simulink model "EE563TermProjectErencanDuymaz"  (R2013a)
settings: Solver=ode4  StartTime=0.0  StopTime=2  FixedStep=1/25600  RelTol=1e-3
libraries: powerlib_meascontrol x44, simulink x8, powerlib x1
settings Model: Creator=Eren  LastModifiedBy=Eren

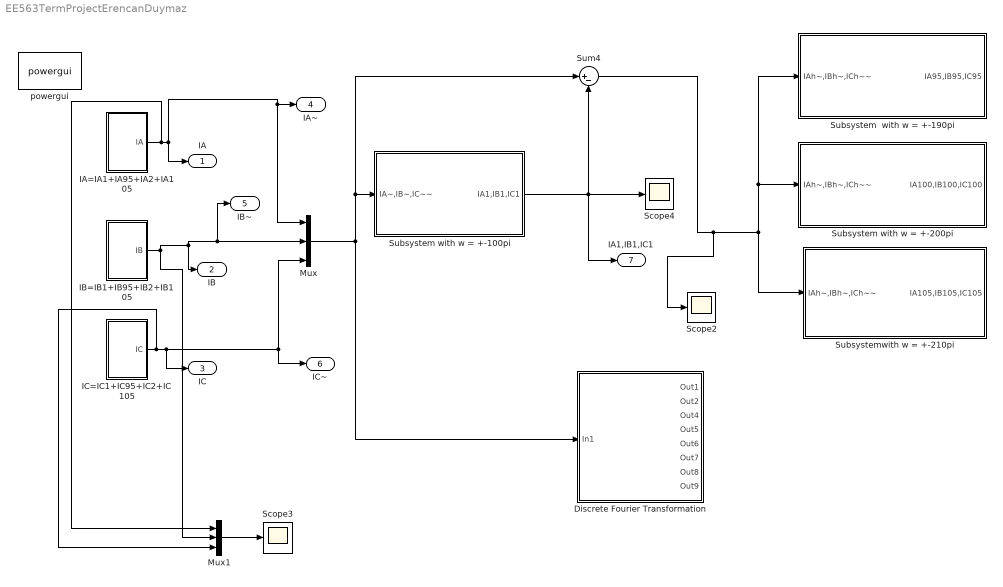
== system EE563TermProjectErencanDuymaz ==
  Discrete Fourier Transformation : Subsystem
  "IA=IA1+IA95+IA2+IA105 " : Subsystem
  "IB=IB1+IB95+IB2+IB105 " : Subsystem
  "IC=IC1+IC95+IC2+IC105 " : Subsystem
  Mux : Mux  Inputs=3
  Mux1 : Mux  Inputs=3
  Scope2 : Scope
      settings: YMin=-1000  YMax=1000  SaveName=ScopeData5
  Scope3 : Scope
      settings: TimeRange=0.2005801931657021  YMin=-3000  YMax=3000  SaveName=ScopeData8
  Scope4 : Scope
      settings: YMin=-3000  YMax=3000  SaveName=ScopeData7
  Subsystem  with w = +-190pi : Subsystem
  Subsystem with w = +-100pi : Subsystem
  Subsystem with w = +-200pi : Subsystem
  "Subsystemwith w = +-210pi " : Subsystem
  Sum4 : Sum  Inputs=|+-
  powergui : powerlib/powergui  Priority=1  SimulationMode=Continuous  SolverType=Tustin  SampleTime=50e-6  frequency=60  SPID=off  DisableSnubberDevices=off  DisableRonSwitches=off  DisableVfSwitches=off  SwTol=0  Interpol=off  DisplayEquations=off  frequencyindice=50  Pbase=100e6  ErrMax=1e-4  Iterations=50  UnitsV=kV  UnitsW=MW  FunctionMessages=off  echomessages=off  HookPort=off  EnableUseOfTLC=off  x0status=blocks  RestoreLinks=warning  ResistiveCurrentMeasurement=off  Frange=[0:2:500]  Ylog=off  Xlog=on  ShowGrid=off  save=off  variable=ZData  ZoomFFT=off  StartTime=0.0  cycles=1  DisplayStyle=1  fundamental=60  FreqAxis=off  MaxFrequency=1000  frequencyindicesteady=1  RmsSteady=1  display=off  Ts=0  methode=off
  IA : Outport
  "IB " : Outport  Port=2
  "IC " : Outport  Port=3
  "IA~ " : Outport  Port=4
  IB~ : Outport  Port=5
  IC~ : Outport  Port=6
  IA1,IB1,IC1 : Outport  Port=7
  wires:
  "IA=IA1+IA95+IA2+IA105 "/1(IA) -> Mux1/1, Mux/1, "IA~ "/1, IA/1
  "IB=IB1+IB95+IB2+IB105 "/1("IB ") -> Mux/2, IB~/1, "IB "/1, Mux1/2
  "IC=IC1+IC95+IC2+IC105 "/1("IC ") -> Mux1/3, "IC "/1, Mux/3, IC~/1
  Mux/1 -> Sum4/1, Subsystem with w = +-100pi/1(IA~,IB~,IC~~), Discrete Fourier Transformation/1(In1)
  Subsystem with w = +-100pi/1(IA1,IB1,IC1) -> Scope4/1, IA1,IB1,IC1/1, Sum4/2
  Sum4/1 -> Subsystem  with w = +-190pi/1(IAh~,IBh~,ICh~~), Subsystem with w = +-200pi/1(IAh~,IBh~,ICh~~), "Subsystemwith w = +-210pi "/1(IAh~,IBh~,ICh~~), Scope2/1
  Mux1/1 -> Scope3/1

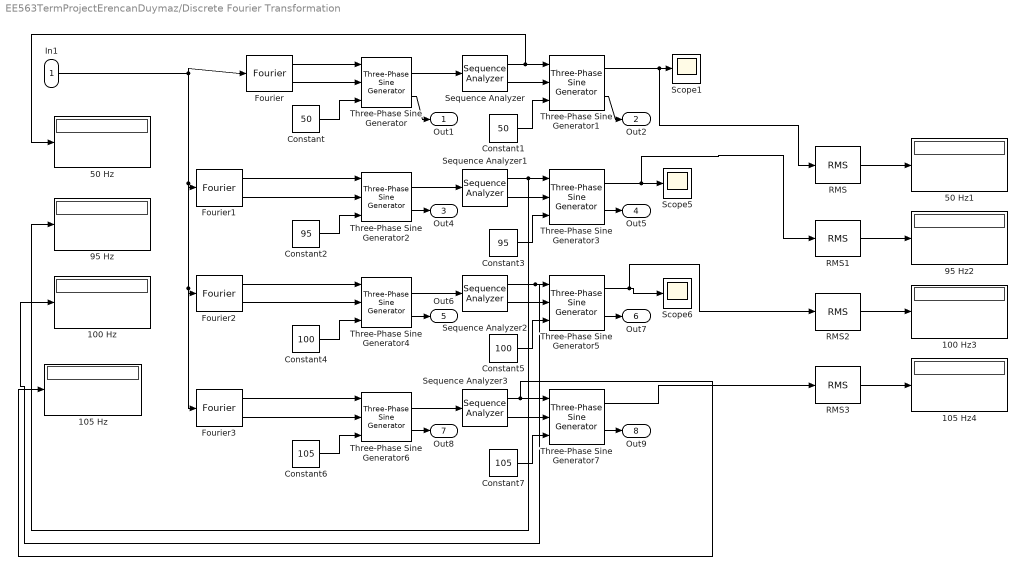
== system EE563TermProjectErencanDuymaz/Discrete Fourier Transformation ==
  In1 : Inport
  100 Hz : Display
  100 Hz3 : Display
  105 Hz : Display
  105 Hz4 : Display
  50 Hz : Display
  50 Hz1 : Display
  "95 Hz " : Display
  95 Hz2 : Display
  Constant : Constant  Value=50
  Constant1 : Constant  Value=50
  Constant2 : Constant  Value=95
  Constant3 : Constant  Value=95
  Constant4 : Constant  Value=100
  Constant5 : Constant  Value=100
  Constant6 : Constant  Value=105
  Constant7 : Constant  Value=105
  Fourier : powerlib_meascontrol/Measurements/Fourier  Freq=5  n=10  InInit=[0, 0]  Ts=0
  Fourier1 : powerlib_meascontrol/Measurements/Fourier  Freq=5  n=19  InInit=[0, 0]  Ts=0
  Fourier2 : powerlib_meascontrol/Measurements/Fourier  Freq=5  n=20  InInit=[0, 0]  Ts=0
  Fourier3 : powerlib_meascontrol/Measurements/Fourier  Freq=5  n=21  InInit=[0, 0]  Ts=0
  RMS : powerlib_meascontrol/Measurements/RMS  TrueRMS=on  Freq=50  RMSInit=120  Ts=0
  RMS1 : powerlib_meascontrol/Measurements/RMS  TrueRMS=on  Freq=95  RMSInit=120  Ts=0
  RMS2 : powerlib_meascontrol/Measurements/RMS  TrueRMS=on  Freq=100  RMSInit=120  Ts=0
  RMS3 : powerlib_meascontrol/Measurements/RMS  TrueRMS=on  Freq=105  RMSInit=120  Ts=0
  Scope1 : Scope
      settings: YMin=-3000  YMax=3000
  Scope5 : Scope
      settings: YMin=-150  YMax=150
  Scope6 : Scope
      settings: YMin=-120  YMax=120  SaveName=ScopeData9
  Sequence Analyzer : powerlib_meascontrol/Measurements/Sequence Analyzer  Freq=5  n=10  seq=Positive Negative Zero  InInit=[0, 0]  Ts=0
  Sequence Analyzer1 : powerlib_meascontrol/Measurements/Sequence Analyzer  Freq=5  n=19  seq=Positive Negative Zero  InInit=[0, 0]  Ts=0
  Sequence Analyzer2 : powerlib_meascontrol/Measurements/Sequence Analyzer  Freq=5  n=20  seq=Positive Negative Zero  InInit=[0, 0]  Ts=0
  Sequence Analyzer3 : powerlib_meascontrol/Measurements/Sequence Analyzer  Freq=5  n=21  seq=Positive Negative Zero  InInit=[0, 0]  Ts=0
  Three-Phase Sine Generator{,1..7} (8 alike) : powerlib_meascontrol/Pulse & Signal Generators/Three-Phase Sine Generator  Ts=0
  Out1 : Outport
  Out2 : Outport  Port=2
  Out4 : Outport  Port=3
  Out5 : Outport  Port=4
  Out6 : Outport  Port=5
  Out7 : Outport  Port=6
  Out8 : Outport  Port=7
  Out9 : Outport  Port=8
  wires:
  Three-Phase Sine Generator1/1 -> RMS/1, Scope1/1
  Three-Phase Sine Generator7/2 -> Out9/1
  Three-Phase Sine Generator1/2 -> Out2/1
  Three-Phase Sine Generator2/2 -> Out4/1
  Three-Phase Sine Generator5/2 -> Out7/1
  Three-Phase Sine Generator6/2 -> Out8/1
  Three-Phase Sine Generator3/2 -> Out5/1
  Three-Phase Sine Generator/2 -> Out1/1
  Three-Phase Sine Generator4/2 -> Out6/1
  Fourier2/1 -> Three-Phase Sine Generator4/1
  Fourier3/1 -> Three-Phase Sine Generator6/1
  Sequence Analyzer1/1 -> "95 Hz "/1, Three-Phase Sine Generator3/1
  Three-Phase Sine Generator4/1 -> Sequence Analyzer2/1
  Fourier/2 -> Three-Phase Sine Generator/2
  Sequence Analyzer/2 -> Three-Phase Sine Generator1/2
  Constant1/1 -> Three-Phase Sine Generator1/3
  Three-Phase Sine Generator6/1 -> Sequence Analyzer3/1
  Sequence Analyzer3/2 -> Three-Phase Sine Generator7/2
  Fourier2/2 -> Three-Phase Sine Generator4/2
  Fourier1/2 -> Three-Phase Sine Generator2/2
  Three-Phase Sine Generator2/1 -> Sequence Analyzer1/1
  Fourier3/2 -> Three-Phase Sine Generator6/2
  Sequence Analyzer/1 -> 50 Hz/1, Three-Phase Sine Generator1/1
  Sequence Analyzer1/2 -> Three-Phase Sine Generator3/2
  Constant2/1 -> Three-Phase Sine Generator2/3
  Sequence Analyzer2/1 -> 100 Hz/1, Three-Phase Sine Generator5/1
  Sequence Analyzer2/2 -> Three-Phase Sine Generator5/2
  Constant4/1 -> Three-Phase Sine Generator4/3
  Constant5/1 -> Three-Phase Sine Generator5/3
  Three-Phase Sine Generator5/1 -> RMS2/1, Scope6/1
  Constant/1 -> Three-Phase Sine Generator/3
  Three-Phase Sine Generator/1 -> Sequence Analyzer/1
  Constant3/1 -> Three-Phase Sine Generator3/3
  Constant7/1 -> Three-Phase Sine Generator7/3
  Three-Phase Sine Generator7/1 -> RMS3/1
  Constant6/1 -> Three-Phase Sine Generator6/3
  Three-Phase Sine Generator3/1 -> RMS1/1, Scope5/1
  Fourier1/1 -> Three-Phase Sine Generator2/1
  In1/1 -> Fourier/1, Fourier3/1, Fourier2/1, Fourier1/1
  Fourier/1 -> Three-Phase Sine Generator/1
  Sequence Analyzer3/1 -> 105 Hz/1, Three-Phase Sine Generator7/1
  RMS/1 -> 50 Hz1/1
  RMS1/1 -> 95 Hz2/1
  RMS2/1 -> 100 Hz3/1
  RMS3/1 -> 105 Hz4/1

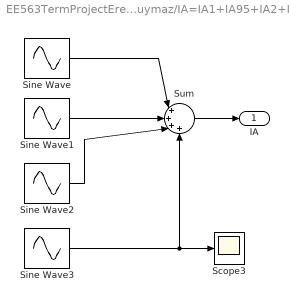
== system EE563TermProjectErencanDuymaz/IA=IA1+IA95+IA2+IA105  ==
  Scope3 : Scope
      settings: TimeRange=0.2005801931657021  YMin=-275  YMax=275  SaveName=ScopeData16
  Sine Wave : Sin  Amplitude=1750*sqrt(2)  Frequency=100*pi  SampleTime=0  VectorParams1D=off
  Sine Wave1 : Sin  Amplitude=190*sqrt(2)  Frequency=190*pi  SampleTime=0  VectorParams1D=off
  Sine Wave2 : Sin  Amplitude=154*sqrt(2)  Frequency=200*pi  SampleTime=0  VectorParams1D=off
  Sine Wave3 : Sin  Amplitude=180*sqrt(2)  Frequency=210*pi  SampleTime=0  VectorParams1D=off
  Sum : Sum  Inputs=|++++
  IA : Outport
  wires:
  Sum/1 -> IA/1
  Sine Wave2/1 -> Sum/3
  Sine Wave/1 -> Sum/1
  Sine Wave3/1 -> Scope3/1, Sum/4
  Sine Wave1/1 -> Sum/2

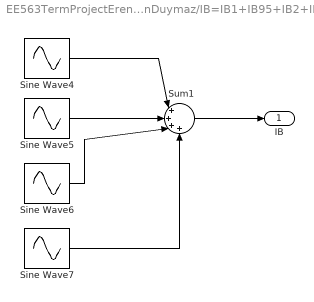
== system EE563TermProjectErencanDuymaz/IB=IB1+IB95+IB2+IB105  ==
  Sine Wave4 : Sin  Amplitude=1261.9*sqrt(2)  Frequency=100*pi  Phase=-0.7439*pi  SampleTime=0  VectorParams1D=off
  Sine Wave5 : Sin  Amplitude=95.4*sqrt(2)  Frequency=190*pi  Phase=-0.9711*pi  SampleTime=0  VectorParams1D=off
  Sine Wave6 : Sin  Amplitude=77.95*sqrt(2)  Frequency=200*pi  Phase=-0.9503*pi  SampleTime=0  VectorParams1D=off
  Sine Wave7 : Sin  Amplitude=96.4*sqrt(2)  Frequency=210*pi  Phase=-0.883*pi  SampleTime=0  VectorParams1D=off
  Sum1 : Sum  Inputs=|++++
  "IB " : Outport
  wires:
  Sum1/1 -> "IB "/1
  Sine Wave5/1 -> Sum1/2
  Sine Wave4/1 -> Sum1/1
  Sine Wave6/1 -> Sum1/3
  Sine Wave7/1 -> Sum1/4

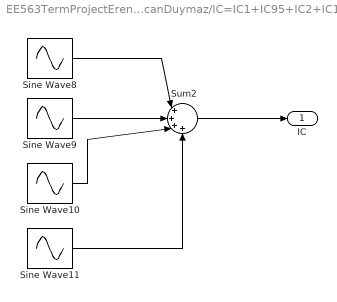
== system EE563TermProjectErencanDuymaz/IC=IC1+IC95+IC2+IC105  ==
  Sine Wave10 : Sin  Amplitude=77.95*sqrt(2)  Frequency=200*pi  Phase=0.9503*pi  SampleTime=0  VectorParams1D=off
  Sine Wave11 : Sin  Amplitude=96.4*sqrt(2)  Frequency=210*pi  Phase=0.883*pi  SampleTime=0  VectorParams1D=off
  Sine Wave8 : Sin  Amplitude=1261.9*sqrt(2)  Frequency=100*pi  Phase=0.7439*pi  SampleTime=0  VectorParams1D=off
  Sine Wave9 : Sin  Amplitude=95.4*sqrt(2)  Frequency=190*pi  Phase=0.9711*pi  SampleTime=0  VectorParams1D=off
  Sum2 : Sum  Inputs=|++++
  "IC " : Outport
  wires:
  Sine Wave11/1 -> Sum2/4
  Sine Wave10/1 -> Sum2/3
  Sine Wave9/1 -> Sum2/2
  Sine Wave8/1 -> Sum2/1
  Sum2/1 -> "IC "/1

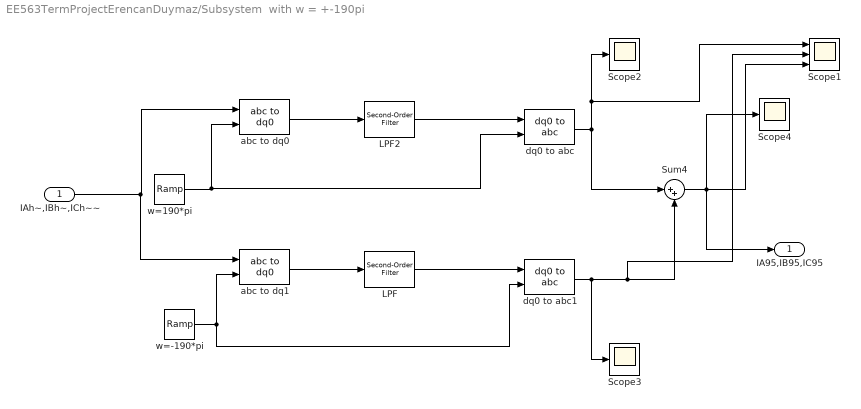
== system EE563TermProjectErencanDuymaz/Subsystem  with w = +-190pi ==
  IAh~,IBh~,ICh~~ : Inport
  LPF : powerlib_meascontrol/Filters/Second-Order Filter  FilterType=Lowpass  Fo=2.5  Zeta=0.707  Ts=0  Initialize=on  Vac_Init="[0,  0,  60]"  Vdc_Init=0  PlotResponse=off  FreqRange=[0, 500, 1]
  "LPF2 " : powerlib_meascontrol/Filters/Second-Order Filter  FilterType=Lowpass  Fo=2.5  Zeta=0.707  Ts=0  Initialize=on  Vac_Init="[0,  0,  60]"  Vdc_Init=0  PlotResponse=off  FreqRange=[0, 500, 1]
  Scope1 : Scope  NumInputPorts=3
      settings: YMin=32.5~-5~-5  YMax=60~5~5  SaveName=ScopeData10
  Scope2 : Scope
      settings: YMin=-3000  YMax=3000  SaveName=ScopeData2
  Scope3 : Scope
      settings: YMin=-3000  YMax=3000  SaveName=ScopeData3
  Scope4 : Scope
      settings: YMin=-3000  YMax=3000  SaveName=ScopeData4
  Sum4 : Sum  Inputs=|++
  abc to dq0 : powerlib_meascontrol/Transformations/abc to dq0  Alignment=90 degrees behind phase A axis
  abc to dq1 : powerlib_meascontrol/Transformations/abc to dq0  Alignment=90 degrees behind phase A axis
  dq0 to abc : powerlib_meascontrol/Transformations/dq0 to abc  Alignment=90 degrees behind phase A axis
  dq0 to abc1 : powerlib_meascontrol/Transformations/dq0 to abc  Alignment=90 degrees behind phase A axis
  "w=-190*pi " : simulink/Sources/Ramp  slope=-190*pi  start=0  X0=0
  "w=190*pi " : simulink/Sources/Ramp  slope=190*pi  start=0  X0=0
  "IA95,IB95,IC95 " : Outport
  wires:
  Sum4/1 -> Scope1/3, "IA95,IB95,IC95 "/1, Scope4/1
  dq0 to abc1/1 -> Scope1/2, Sum4/2, Scope3/1
  abc to dq1/1 -> LPF/1
  abc to dq0/1 -> "LPF2 "/1
  "LPF2 "/1 -> dq0 to abc/1
  LPF/1 -> dq0 to abc1/1
  IAh~,IBh~,ICh~~/1 -> abc to dq1/1, abc to dq0/1
  "w=190*pi "/1 -> dq0 to abc/2, abc to dq0/2
  "w=-190*pi "/1 -> abc to dq1/2, dq0 to abc1/2
  dq0 to abc/1 -> Sum4/1, Scope1/1, Scope2/1

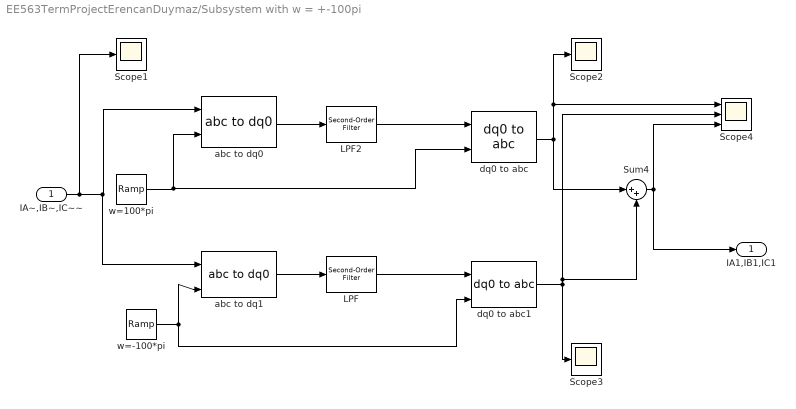
== system EE563TermProjectErencanDuymaz/Subsystem with w = +-100pi ==
  IA~,IB~,IC~~ : Inport
  LPF : powerlib_meascontrol/Filters/Second-Order Filter  FilterType=Lowpass  Fo=2.5  Zeta=0.707  Ts=0  Initialize=on  Vac_Init="[0,  0,  60]"  Vdc_Init=0  PlotResponse=off  FreqRange=[0, 500, 1]
  "LPF2 " : powerlib_meascontrol/Filters/Second-Order Filter  FilterType=Lowpass  Fo=2.5  Zeta=0.707  Ts=0  Initialize=on  Vac_Init="[0,  0,  60]"  Vdc_Init=0  PlotResponse=off  FreqRange=[0, 500, 1]
  Scope1 : Scope
      settings: TimeRange=0.2014563939396098  YMin=-3000  YMax=3000  SaveName=ScopeData6
  Scope2 : Scope
      settings: YMin=-3000  YMax=3000  SaveName=ScopeData2
  Scope3 : Scope
      settings: YMin=-3000  YMax=3000  SaveName=ScopeData3
  Scope4 : Scope  NumInputPorts=3
      settings: TimeRange=0.200993419768845  YMin=-3000~-750~-3000  YMax=3000~750~3000  SaveName=ScopeData4
  Sum4 : Sum  Inputs=|++
  abc to dq0 : powerlib_meascontrol/Transformations/abc to dq0  Alignment=90 degrees behind phase A axis
  abc to dq1 : powerlib_meascontrol/Transformations/abc to dq0  Alignment=90 degrees behind phase A axis
  dq0 to abc : powerlib_meascontrol/Transformations/dq0 to abc  Alignment=90 degrees behind phase A axis
  dq0 to abc1 : powerlib_meascontrol/Transformations/dq0 to abc  Alignment=90 degrees behind phase A axis
  "w=-100*pi " : simulink/Sources/Ramp  slope=-100*pi  start=0  X0=0
  "w=100*pi " : simulink/Sources/Ramp  slope=100*pi  start=0  X0=0
  IA1,IB1,IC1 : Outport
  wires:
  Sum4/1 -> Scope4/3, IA1,IB1,IC1/1
  dq0 to abc1/1 -> Scope4/2, Sum4/2, Scope3/1
  dq0 to abc/1 -> Scope4/1, Scope2/1, Sum4/1
  abc to dq1/1 -> LPF/1
  abc to dq0/1 -> "LPF2 "/1
  "LPF2 "/1 -> dq0 to abc/1
  LPF/1 -> dq0 to abc1/1
  IA~,IB~,IC~~/1 -> Scope1/1, abc to dq1/1, abc to dq0/1
  "w=100*pi "/1 -> dq0 to abc/2, abc to dq0/2
  "w=-100*pi "/1 -> abc to dq1/2, dq0 to abc1/2

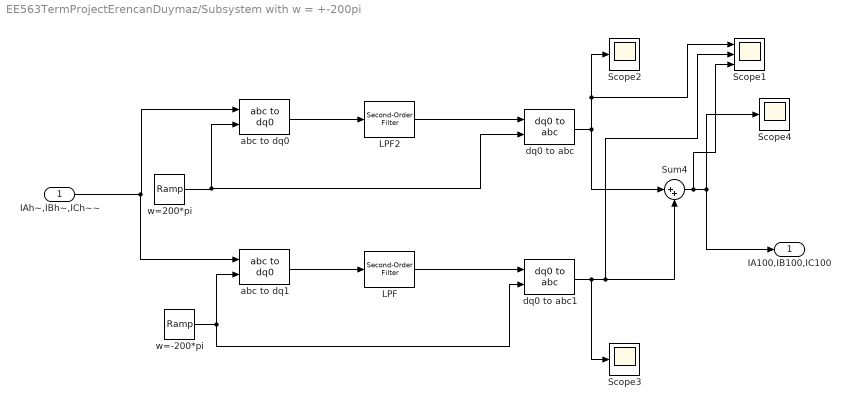
== system EE563TermProjectErencanDuymaz/Subsystem with w = +-200pi ==
  IAh~,IBh~,ICh~~ : Inport
  LPF : powerlib_meascontrol/Filters/Second-Order Filter  FilterType=Lowpass  Fo=2.5  Zeta=0.707  Ts=0  Initialize=on  Vac_Init="[0,  0,  60]"  Vdc_Init=0  PlotResponse=off  FreqRange=[0, 500, 1]
  "LPF2 " : powerlib_meascontrol/Filters/Second-Order Filter  FilterType=Lowpass  Fo=2.5  Zeta=0.707  Ts=0  Initialize=on  Vac_Init="[0,  0,  60]"  Vdc_Init=0  PlotResponse=off  FreqRange=[0, 500, 1]
  Scope1 : Scope  NumInputPorts=3
      settings: YMin=-100~-70~-5  YMax=125~90~5  SaveName=ScopeData11
  Scope2 : Scope
      settings: YMin=-3000  YMax=3000  SaveName=ScopeData2
  Scope3 : Scope
      settings: YMin=-3000  YMax=3000  SaveName=ScopeData3
  Scope4 : Scope
      settings: YMin=-3000  YMax=3000  SaveName=ScopeData4
  Sum4 : Sum  Inputs=|++
  abc to dq0 : powerlib_meascontrol/Transformations/abc to dq0  Alignment=90 degrees behind phase A axis
  abc to dq1 : powerlib_meascontrol/Transformations/abc to dq0  Alignment=90 degrees behind phase A axis
  dq0 to abc : powerlib_meascontrol/Transformations/dq0 to abc  Alignment=90 degrees behind phase A axis
  dq0 to abc1 : powerlib_meascontrol/Transformations/dq0 to abc  Alignment=90 degrees behind phase A axis
  "w=-200*pi " : simulink/Sources/Ramp  slope=-200*pi  start=0  X0=0
  "w=200*pi " : simulink/Sources/Ramp  slope=200*pi  start=0  X0=0
  "IA100,IB100,IC100 " : Outport
  wires:
  Sum4/1 -> Scope1/3, "IA100,IB100,IC100 "/1, Scope4/1
  dq0 to abc1/1 -> Scope1/2, Sum4/2, Scope3/1
  abc to dq1/1 -> LPF/1
  abc to dq0/1 -> "LPF2 "/1
  "LPF2 "/1 -> dq0 to abc/1
  LPF/1 -> dq0 to abc1/1
  IAh~,IBh~,ICh~~/1 -> abc to dq1/1, abc to dq0/1
  "w=200*pi "/1 -> dq0 to abc/2, abc to dq0/2
  "w=-200*pi "/1 -> abc to dq1/2, dq0 to abc1/2
  dq0 to abc/1 -> Sum4/1, Scope1/1, Scope2/1

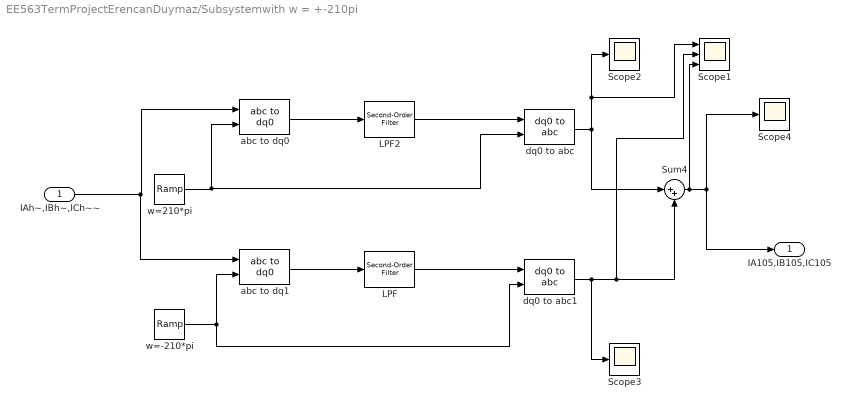
== system EE563TermProjectErencanDuymaz/Subsystemwith w = +-210pi  ==
  IAh~,IBh~,ICh~~ : Inport
  LPF : powerlib_meascontrol/Filters/Second-Order Filter  FilterType=Lowpass  Fo=2.5  Zeta=0.707  Ts=0  Initialize=on  Vac_Init="[0,  0,  60]"  Vdc_Init=0  PlotResponse=off  FreqRange=[0, 500, 1]
  "LPF2 " : powerlib_meascontrol/Filters/Second-Order Filter  FilterType=Lowpass  Fo=2.5  Zeta=0.707  Ts=0  Initialize=on  Vac_Init="[0,  0,  60]"  Vdc_Init=0  PlotResponse=off  FreqRange=[0, 500, 1]
  Scope1 : Scope  NumInputPorts=3
      settings: YMin=-100~-50~-5  YMax=100~50~5  SaveName=ScopeData12
  Scope2 : Scope
      settings: YMin=-3000  YMax=3000  SaveName=ScopeData2
  Scope3 : Scope
      settings: YMin=-3000  YMax=3000  SaveName=ScopeData3
  Scope4 : Scope
      settings: YMin=-3000  YMax=3000  SaveName=ScopeData4
  Sum4 : Sum  Inputs=|++
  abc to dq0 : powerlib_meascontrol/Transformations/abc to dq0  Alignment=90 degrees behind phase A axis
  abc to dq1 : powerlib_meascontrol/Transformations/abc to dq0  Alignment=90 degrees behind phase A axis
  dq0 to abc : powerlib_meascontrol/Transformations/dq0 to abc  Alignment=90 degrees behind phase A axis
  dq0 to abc1 : powerlib_meascontrol/Transformations/dq0 to abc  Alignment=90 degrees behind phase A axis
  "w=-210*pi " : simulink/Sources/Ramp  slope=-210*pi  start=0  X0=0
  "w=210*pi " : simulink/Sources/Ramp  slope=210*pi  start=0  X0=0
  "IA105,IB105,IC105 " : Outport
  wires:
  Sum4/1 -> Scope1/3, "IA105,IB105,IC105 "/1, Scope4/1
  dq0 to abc1/1 -> Scope1/2, Sum4/2, Scope3/1
  dq0 to abc/1 -> Sum4/1, Scope1/1, Scope2/1
  abc to dq1/1 -> LPF/1
  abc to dq0/1 -> "LPF2 "/1
  "LPF2 "/1 -> dq0 to abc/1
  LPF/1 -> dq0 to abc1/1
  IAh~,IBh~,ICh~~/1 -> abc to dq1/1, abc to dq0/1
  "w=210*pi "/1 -> dq0 to abc/2, abc to dq0/2
  "w=-210*pi "/1 -> abc to dq1/2, dq0 to abc1/2
